simulink model "koen_three_shunt_sampling_model"  (R2024b)
settings: Solver=FixedStepDiscrete  StartTime=0.0  StopTime=0.02  FixedStep=6.25e-05  RelTol=1e-3
PreLoadFcn:
  | FOC_PWM_HALF_ARR=2655; SAMPLE_MARGIN=120; SAMPLE_LEFT_LIMIT=(FOC_PWM_HALF_ARR-SAMPLE_MARGIN); SAMPLE_RIGHT_LIMIT=(FOC_PWM_HALF_ARR+SAMPLE_MARGIN);
libraries: simulink x6
settings Model: Creator=10095  LastModifiedBy=10095

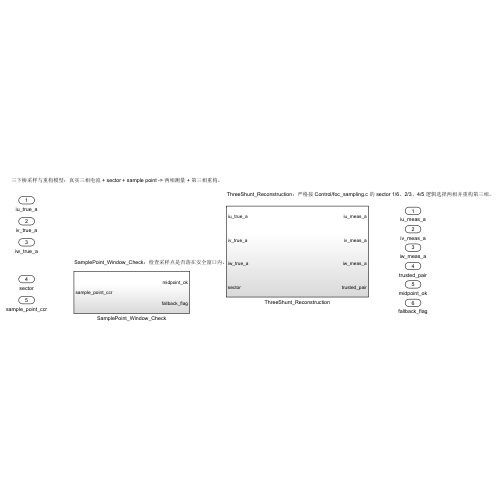
[thumbnail: Simulink's stored preview of the top-level diagram]
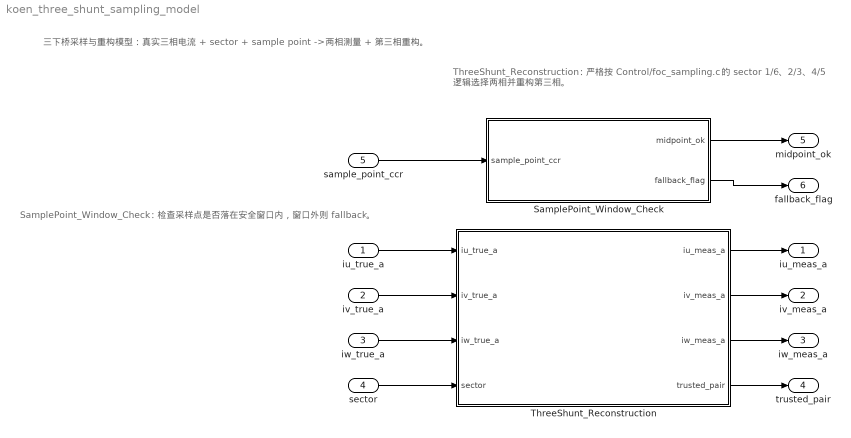
== system koen_three_shunt_sampling_model ==
  note: SamplePoint_Window_Check：检查采样点是否落在安全窗口内，窗口外则 fallback。
  note: ThreeShunt_Reconstruction：严格按 Control/foc_sampling.c 的 sector 1/6、2/3、4/5 逻辑选择两相并重构第三相。
  note: 三下桥采样与重构模型：真实三相电流 + sector + sample point -> 两相测量 + 第三相重构。
  iu_true_a : Inport
  iv_true_a : Inport  Port=2
  iw_true_a : Inport  Port=3
  sector : Inport  Port=4
  sample_point_ccr : Inport  Port=5
  SamplePoint_Window_Check : Subsystem  Description=SamplePoint_Window_Check：检查采样点是否落在安全窗口内，窗口外则 fallback。
  ThreeShunt_Reconstruction : Subsystem  Description=ThreeShunt_Reconstruction：严格按 Control/foc_sampling.c 的 sector 1/6、2/3、4/5 逻辑选择两相并重构第三相。
  iu_meas_a : Outport
  iv_meas_a : Outport  Port=2
  iw_meas_a : Outport  Port=3
  trusted_pair : Outport  Port=4
  midpoint_ok : Outport  Port=5
  fallback_flag : Outport  Port=6
  wires:
  sector/1 -> ThreeShunt_Reconstruction/4(sector)
  sample_point_ccr/1 -> SamplePoint_Window_Check/1(sample_point_ccr)
  iu_true_a/1 -> ThreeShunt_Reconstruction/1(iu_true_a)
  iw_true_a/1 -> ThreeShunt_Reconstruction/3(iw_true_a)
  iv_true_a/1 -> ThreeShunt_Reconstruction/2(iv_true_a)
  SamplePoint_Window_Check/2(fallback_flag) -> fallback_flag/1
  SamplePoint_Window_Check/1(midpoint_ok) -> midpoint_ok/1
  ThreeShunt_Reconstruction/1(iu_meas_a) -> iu_meas_a/1
  ThreeShunt_Reconstruction/2(iv_meas_a) -> iv_meas_a/1
  ThreeShunt_Reconstruction/3(iw_meas_a) -> iw_meas_a/1
  ThreeShunt_Reconstruction/4(trusted_pair) -> trusted_pair/1

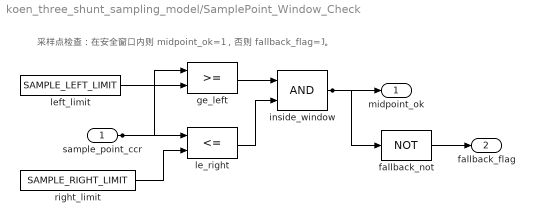
== system koen_three_shunt_sampling_model/SamplePoint_Window_Check ==
  note: 采样点检查：在安全窗口内则 midpoint_ok=1，否则 fallback_flag=1。
  sample_point_ccr : Inport
  fallback_not : Logic  Operator=NOT  AllPortsSameDT=off  OutDataTypeStr=boolean
  ge_left : RelationalOperator  OutDataTypeStr=boolean  RndMeth=Simplest  InputSameDT=off
  inside_window : Logic  AllPortsSameDT=off  OutDataTypeStr=boolean
  le_right : RelationalOperator  Operator=<=  OutDataTypeStr=boolean  RndMeth=Simplest  InputSameDT=off
  left_limit : Constant  Value=SAMPLE_LEFT_LIMIT
  right_limit : Constant  Value=SAMPLE_RIGHT_LIMIT
  midpoint_ok : Outport
  fallback_flag : Outport  Port=2
  wires:
  left_limit/1 -> ge_left/2
  sample_point_ccr/1 -> ge_left/1, le_right/1
  right_limit/1 -> le_right/2
  ge_left/1 -> inside_window/1
  le_right/1 -> inside_window/2
  fallback_not/1 -> fallback_flag/1
  inside_window/1 -> midpoint_ok/1, fallback_not/1

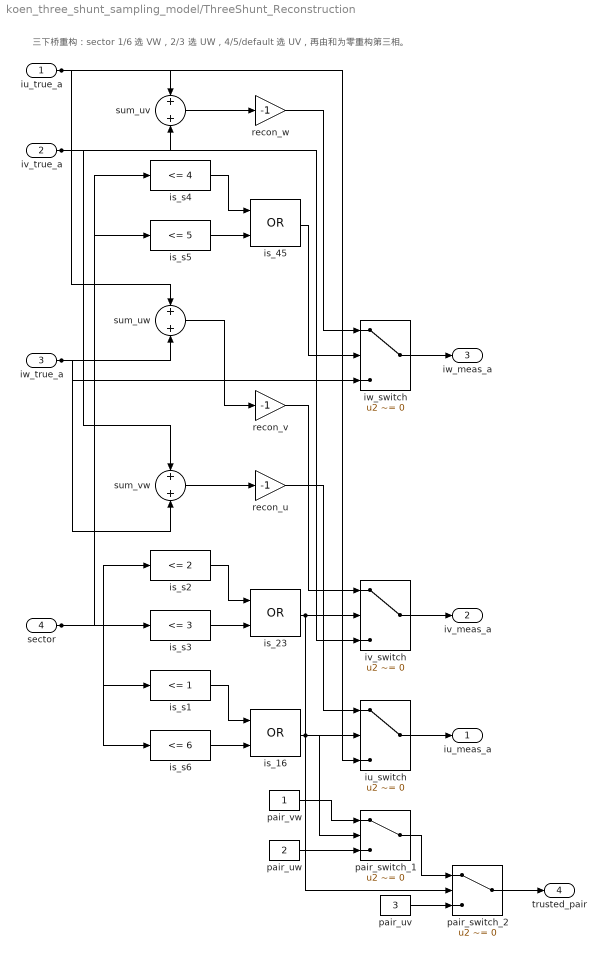
== system koen_three_shunt_sampling_model/ThreeShunt_Reconstruction ==
  note: 三下桥重构：sector 1/6 选 VW，2/3 选 UW，4/5/default 选 UV，再由和为零重构第三相。
  iu_true_a : Inport
  iv_true_a : Inport  Port=2
  iw_true_a : Inport  Port=3
  sector : Inport  Port=4
  is_16 : Logic  Operator=OR  AllPortsSameDT=off  OutDataTypeStr=boolean
  is_23 : Logic  Operator=OR  AllPortsSameDT=off  OutDataTypeStr=boolean
  is_45 : Logic  Operator=OR  AllPortsSameDT=off  OutDataTypeStr=boolean
  is_s1 : simulink/Logic and Bit Operations/Compare To Constant  relop=<=  const=1  OutDataTypeStr=boolean
  is_s2 : simulink/Logic and Bit Operations/Compare To Constant  relop=<=  const=2  OutDataTypeStr=boolean
  is_s3 : simulink/Logic and Bit Operations/Compare To Constant  relop=<=  const=3  OutDataTypeStr=boolean
  is_s4 : simulink/Logic and Bit Operations/Compare To Constant  relop=<=  const=4  OutDataTypeStr=boolean
  is_s5 : simulink/Logic and Bit Operations/Compare To Constant  relop=<=  const=5  OutDataTypeStr=boolean
  is_s6 : simulink/Logic and Bit Operations/Compare To Constant  relop=<=  const=6  OutDataTypeStr=boolean
  iu_switch : Switch  Criteria=u2 ~= 0  Threshold=0.5  SaturateOnIntegerOverflow=off  InputSameDT=off
  iv_switch : Switch  Criteria=u2 ~= 0  Threshold=0.5  SaturateOnIntegerOverflow=off  InputSameDT=off
  iw_switch : Switch  Criteria=u2 ~= 0  Threshold=0.5  SaturateOnIntegerOverflow=off  InputSameDT=off
  pair_switch_1 : Switch  Criteria=u2 ~= 0  Threshold=0.5  SaturateOnIntegerOverflow=off  InputSameDT=off
  pair_switch_2 : Switch  Criteria=u2 ~= 0  Threshold=0.5  SaturateOnIntegerOverflow=off  InputSameDT=off
  pair_uv : Constant  Value=3
  pair_uw : Constant  Value=2
  pair_vw : Constant
  recon_u : Gain  Gain=-1
  recon_v : Gain  Gain=-1
  recon_w : Gain  Gain=-1
  sum_uv : Sum
  sum_uw : Sum
  sum_vw : Sum
  iu_meas_a : Outport
  iv_meas_a : Outport  Port=2
  iw_meas_a : Outport  Port=3
  trusted_pair : Outport  Port=4
  wires:
  is_s1/1 -> is_16/1
  iu_true_a/1 -> sum_uw/1, sum_uv/1, iu_switch/3
  iv_true_a/1 -> sum_vw/1, sum_uv/2, iv_switch/3
  pair_switch_2/1 -> trusted_pair/1
  iw_switch/1 -> iw_meas_a/1
  iw_true_a/1 -> sum_vw/2, sum_uw/2, iw_switch/3
  is_s4/1 -> is_45/1
  is_s5/1 -> is_45/2
  sector/1 -> is_s1/1, is_s2/1, is_s3/1, is_s4/1, is_s5/1, is_s6/1
  sum_uw/1 -> recon_v/1
  sum_uv/1 -> recon_w/1
  sum_vw/1 -> recon_u/1
  is_s2/1 -> is_23/1
  is_s3/1 -> is_23/2
  is_s6/1 -> is_16/2
  recon_w/1 -> iw_switch/1
  is_16/1 -> iu_switch/2, pair_switch_1/2
  is_45/1 -> iw_switch/2
  recon_v/1 -> iv_switch/1
  iu_switch/1 -> iu_meas_a/1
  recon_u/1 -> iu_switch/1
  is_23/1 -> pair_switch_2/2, iv_switch/2
  pair_vw/1 -> pair_switch_1/1
  pair_uw/1 -> pair_switch_1/3
  pair_switch_1/1 -> pair_switch_2/1
  iv_switch/1 -> iv_meas_a/1
  pair_uv/1 -> pair_switch_2/3
